simulink model "Regulador_Sims"  (R2023b)
settings: Solver=VariableStepAuto  StartTime=0.0  StopTime=0.01  RelTol=1e-3
values from neighbouring files (symbols this model uses):
  C = 10e-6    (= 1e-05)    [CD_CD.m]    (also in Condiciones.mat)
  d = 0.4    [CD_CD.m]    (also in Condiciones.mat)
  d2 = 0.6    [CD_CD.m]    (also in Condiciones.mat)
  L = 2e-3    (= 0.002)    [CD_CD.m]    (also in Condiciones.mat)
  R = 10    [CD_CD.m]    (also in Condiciones.mat)
settings Model: Creator=andre  LastModifiedBy=andre

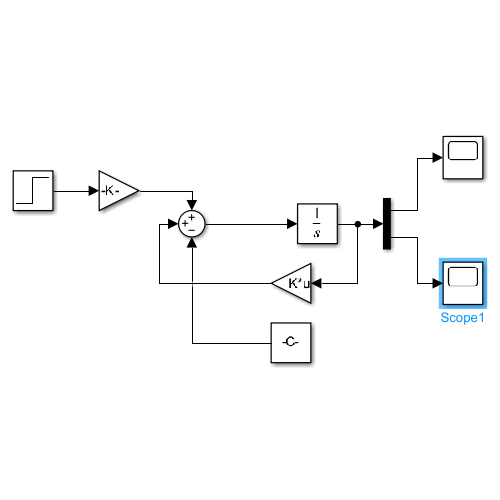
[thumbnail: Simulink's stored preview of the top-level diagram]
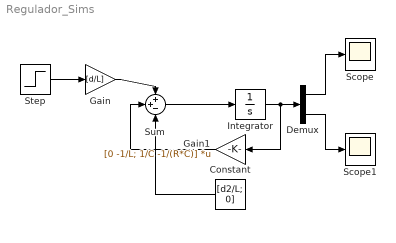
== system Regulador_Sims ==
  Constant : Constant  Value=[d2/L; 0]
  Demux : Demux  Outputs=2
  Gain : Gain  Gain=[d/L]
  Gain1 : Gain  Gain=[0 -1/L; 1/C -1/(R*C)]  Multiplication=Matrix(K*u)
  Integrator : Integrator
  Scope : Scope
  Scope1 : Scope
  Step : Step  Time=0  After=32  SampleTime=0
  Sum : Sum  Inputs=++-
  wires:
  Step/1 -> Gain/1
  Gain/1 -> Sum/1
  Sum/1 -> Integrator/1
  Gain1/1 -> Sum/2
  Integrator/1 -> Demux/1, Gain1/1
  Demux/1 -> Scope/1
  Demux/2 -> Scope1/1
  Constant/1 -> Sum/3
